simulink model "generic"  (R2022b)
settings: Solver=VariableStepAuto  StartTime=0.0  StopTime=inf  RelTol=1e-3
undefined symbols (not defined in the file or in its folder): left_first_line_point_x, right_first_line_point_x, route1_waypoint_raw
libraries: CarMaker4SL x69, slpidlib x3, simulink x1
(part 3 of 4)

== system generic/CarMaker/IPG Vehicle/CarAndTrailer/Forces/Vehicle Forces ==
  Sync_In : Inport
  Bus Creator1 : BusCreator  Inputs=12
  Bus Creator8 : BusCreator  Inputs=16
  BusCreator1 : BusCreator  Inputs=4
  BusCreator2 : BusCreator  Inputs=9
  Demux : Demux  Outputs=16
      settings: DisplayOption=none
  Demux1 : Demux  Outputs=12
      settings: DisplayOption=none
  Demux2 : Demux  Outputs=13
      settings: DisplayOption=none
  Forces : S-Function  FunctionName=CM_Sfun  Parameters='Forces'  SFunctionDeploymentMode=off  EnableBusSupport=off
  Terminator : Terminator
  Sync_Out : Outport  VectorParamsAs1DForOutWhenUnconnected=off
  Car.Virtual : Outport  Port=2  VectorParamsAs1DForOutWhenUnconnected=off
  Car.Aero : Outport  Port=3  VectorParamsAs1DForOutWhenUnconnected=off
  Car.Load : Outport  Port=4  VectorParamsAs1DForOutWhenUnconnected=off
  wires:
  BusCreator1/1 -> Terminator/1  "Aero IF (in)"
  Demux2/13 -> BusCreator2/9  "car Aero Trq_1 z"
  Demux2/12 -> BusCreator2/8  "car Aero Trq_1 y"
  Demux2/11 -> BusCreator2/7  "car Aero Trq_1 x"
  Demux2/10 -> BusCreator2/6  "car Aero Frc_1 z"
  Demux2/9 -> BusCreator2/5  "car Aero Frc_1 y"
  Demux2/8 -> BusCreator2/4  "car Aero Frc_1 x"
  Demux2/7 -> BusCreator2/3  "car Aero PoA_1 z"
  Demux2/6 -> BusCreator2/2  "car Aero PoA_1 y"
  Demux2/5 -> BusCreator2/1  "car Aero PoA_1 x"
  Demux2/4 -> BusCreator1/4  "car Aero tau_1"
  Demux2/3 -> BusCreator1/3  "car Aero ApproachVel_1 z"
  Demux2/2 -> BusCreator1/2  "car Aero ApproachVel_1 y"
  Demux2/1 -> BusCreator1/1  "car Aero ApproachVel_1 x"
  Demux/16 -> Bus Creator8/16  "Car Load_3 tz"
  Demux/15 -> Bus Creator8/15  "Car Load_3 ty"
  Demux/14 -> Bus Creator8/14  "Car Load_3 tx"
  Demux/13 -> Bus Creator8/13  "Car Load_3 mass"
  Demux1/12 -> Bus Creator1/12  "Car Virtual Trq_0 z"
  Demux1/11 -> Bus Creator1/11  "Car Virtual Trq_0 y"
  Demux1/10 -> Bus Creator1/10  "Car Virtual Trq_0 x"
  Demux1/9 -> Bus Creator1/9  "Car Virtual Trq_1 z"
  Demux1/8 -> Bus Creator1/8  "Car Virtual Trq_1 y"
  Demux1/7 -> Bus Creator1/7  "Car Virtual Trq_1 x"
  Demux1/6 -> Bus Creator1/6  "Car Virtual Frc_0 z"
  Demux1/5 -> Bus Creator1/5  "Car Virtual Frc_0 y"
  Demux1/4 -> Bus Creator1/4  "Car Virtual Frc_0 x"
  Sync_In/1 -> Forces/1
  Forces/1 -> Sync_Out/1
  BusCreator2/1 -> Car.Aero/1
  Demux1/1 -> Bus Creator1/1  "Car Virtual Frc_1 x"
  Demux1/2 -> Bus Creator1/2  "Car Virtual Frc_1 y"
  Demux1/3 -> Bus Creator1/3  "Car Virtual Frc_1 z"
  Forces/3 -> Demux2/1
  Forces/2 -> Demux1/1
  Bus Creator1/1 -> Car.Virtual/1
  Bus Creator8/1 -> Car.Load/1
  Demux/1 -> Bus Creator8/1  "Car Load_0 mass"
  Demux/2 -> Bus Creator8/2  "Car Load_0 tx"
  Demux/3 -> Bus Creator8/3  "Car Load_0 ty"
  Demux/4 -> Bus Creator8/4  "Car Load_0 tz"
  Demux/5 -> Bus Creator8/5  "Car Load_1 mass"
  Demux/6 -> Bus Creator8/6  "Car Load_1 tx"
  Demux/7 -> Bus Creator8/7  "Car Load_1 ty"
  Demux/8 -> Bus Creator8/8  "Car Load_1 tz"
  Demux/9 -> Bus Creator8/9  "Car Load_2 mass"
  Demux/10 -> Bus Creator8/10  "Car Load_2 tx"
  Demux/11 -> Bus Creator8/11  "Car Load_2 ty"
  Demux/12 -> Bus Creator8/12  "Car Load_2 tz"
  Forces/4 -> Demux/1

== system generic/CarMaker/IPG Vehicle/CarAndTrailer/Trailer/CreateBus Car.Hitch.FrcTrq ==
  In1 : Inport
  Bus Creator7 : BusCreator  Inputs=6
  Demux7 : Demux  Outputs=6
      settings: DisplayOption=none
  Out1 : Outport  VectorParamsAs1DForOutWhenUnconnected=off
  wires:
  In1/1 -> Demux7/1
  Bus Creator7/1 -> Out1/1
  Demux7/6 -> Bus Creator7/6  "Car Hitch Trq2Car z"
  Demux7/5 -> Bus Creator7/5  "Car Hitch Trq2Car y"
  Demux7/4 -> Bus Creator7/4  "Car Hitch Trq2Car x"
  Demux7/3 -> Bus Creator7/3  "Car Hitch Frc2Car z"
  Demux7/2 -> Bus Creator7/2  "Car Hitch Frc2Car y"
  Demux7/1 -> Bus Creator7/1  "Car Hitch Frc2Car x"

== system generic/CarMaker/IPG Vehicle/CarAndTrailer/Trailer/CreateBus Vhcl.Motion ==
  In1 : Inport
  BusCreator : BusCreator  Inputs=15
  Demux : Demux  Outputs=15
      settings: DisplayOption=none
  Out1 : Outport  VectorParamsAs1DForOutWhenUnconnected=off
  wires:
  Demux/15 -> BusCreator/15  "Vhcl YawAcc"
  Demux/14 -> BusCreator/14  "Vhcl YawVel"
  Demux/13 -> BusCreator/13  "Vhcl Yaw"
  Demux/12 -> BusCreator/12  "Vhcl PitchAcc"
  Demux/11 -> BusCreator/11  "Vhcl PitchVel"
  Demux/10 -> BusCreator/10  "Vhcl Pitch"
  Demux/9 -> BusCreator/9  "Vhcl RollAcc"
  Demux/8 -> BusCreator/8  "Vhcl RollVel"
  Demux/7 -> BusCreator/7  "Vhcl Roll"
  Demux/6 -> BusCreator/6  "Vhcl Hitch_Pos z"
  Demux/5 -> BusCreator/5  "Vhcl Hitch_Pos y"
  Demux/4 -> BusCreator/4  "Vhcl Hitch_Pos x"
  Demux/3 -> BusCreator/3  "Vhcl sRoad"
  Demux/2 -> BusCreator/2  "Vhcl Distance"
  Demux/1 -> BusCreator/1  "Vhcl v"
  In1/1 -> Demux/1
  BusCreator/1 -> Out1/1

== system generic/CarMaker/IPG Vehicle/CarAndTrailer/Trailer/CreateBus Vhcl.PoI ==
  In1 : Inport
  Bus Creator3 : BusCreator  Inputs=18
  Demux3 : Demux  Outputs=18
      settings: DisplayOption=none
  Out1 : Outport  VectorParamsAs1DForOutWhenUnconnected=off
  wires:
  Demux3/18 -> Bus Creator3/18  "Vhcl PoI_GCS Elev"
  Demux3/17 -> Bus Creator3/17  "Vhcl PoI_GCS Lat"
  Demux3/16 -> Bus Creator3/16  "Vhcl PoI_GCS Long"
  Demux3/15 -> Bus Creator3/15  "Vhcl PoI_Acc_1 z"
  Demux3/14 -> Bus Creator3/14  "Vhcl PoI_Acc_1 y"
  Demux3/13 -> Bus Creator3/13  "Vhcl PoI_Acc_1 x"
  Demux3/12 -> Bus Creator3/12  "Vhcl PoI_Vel_1 z"
  Demux3/11 -> Bus Creator3/11  "Vhcl PoI_Vel_1 y"
  Demux3/10 -> Bus Creator3/10  "Vhcl PoI_Vel_1 x"
  Demux3/9 -> Bus Creator3/9  "Vhcl PoI_Acc z"
  Demux3/8 -> Bus Creator3/8  "Vhcl PoI_Acc y"
  Demux3/7 -> Bus Creator3/7  "Vhcl PoI_Acc x"
  Demux3/6 -> Bus Creator3/6  "Vhcl PoI_Vel z"
  Demux3/5 -> Bus Creator3/5  "Vhcl PoI_Vel y"
  Demux3/4 -> Bus Creator3/4  "Vhcl PoI_Vel x"
  Demux3/3 -> Bus Creator3/3  "Vhcl PoI_Pos z"
  Demux3/2 -> Bus Creator3/2  "Vhcl PoI_Pos y"
  In1/1 -> Demux3/1
  Bus Creator3/1 -> Out1/1
  Demux3/1 -> Bus Creator3/1  "Vhcl PoI_Pos x"

== system generic/CarMaker/IPG Vehicle/CarAndTrailer/Trailer/CreateBus Vhcl.Steering ==
  In1 : Inport
  Bus Creator3 : BusCreator  Inputs=4
  Demux : Demux
      settings: DisplayOption=none
  Out1 : Outport  VectorParamsAs1DForOutWhenUnconnected=off
  wires:
  Bus Creator3/1 -> Out1/1
  Demux/1 -> Bus Creator3/1  "Vhcl Steering Ang"
  Demux/3 -> Bus Creator3/3  "Vhcl Steering AngAcc"
  Demux/2 -> Bus Creator3/2  "Vhcl Steering AngVel"
  Demux/4 -> Bus Creator3/4  "Vhcl Steering Trq"
  In1/1 -> Demux/1

== system generic/CarMaker/IPG Vehicle/CarAndTrailer/Trailer/CreateBus Vhcl.Wheel.FL ==
  In1 : Inport
  Bus Creator3 : BusCreator  Inputs=14
  Demux3 : Demux  Outputs=14
      settings: DisplayOption=none
  Out1 : Outport  VectorParamsAs1DForOutWhenUnconnected=off
  wires:
  Demux3/14 -> Bus Creator3/14  "Vhcl Wheel FL Trq_WhlBearing"
  Demux3/13 -> Bus Creator3/13  "Vhcl Wheel FL Trq_T2W"
  Demux3/12 -> Bus Creator3/12  "Vhcl Wheel FL SideSlip"
  Demux3/11 -> Bus Creator3/11  "Vhcl Wheel FL LongSlip"
  Demux3/10 -> Bus Creator3/10  "Vhcl Wheel FL vBelt"
  Demux3/9 -> Bus Creator3/9  "Vhcl Wheel FL Fz"
  Demux3/8 -> Bus Creator3/8  "Vhcl Wheel FL Fy"
  Demux3/7 -> Bus Creator3/7  "Vhcl Wheel FL Fx"
  Demux3/6 -> Bus Creator3/6  "Vhcl Wheel FL r_zxy z"
  Demux3/5 -> Bus Creator3/5  "Vhcl Wheel FL r_zxy y"
  Demux3/4 -> Bus Creator3/4  "Vhcl Wheel FL r_zxy x"
  Demux3/3 -> Bus Creator3/3  "Vhcl Wheel FL t z"
  Demux3/2 -> Bus Creator3/2  "Vhcl Wheel FL t y"
  In1/1 -> Demux3/1
  Bus Creator3/1 -> Out1/1
  Demux3/1 -> Bus Creator3/1  "Vhcl Wheel FL t x"

== system generic/CarMaker/IPG Vehicle/CarAndTrailer/Trailer/CreateBus Vhcl.Wheel.FR ==
  In1 : Inport
  Bus Creator3 : BusCreator  Inputs=14
  Demux3 : Demux  Outputs=14
      settings: DisplayOption=none
  Out1 : Outport  VectorParamsAs1DForOutWhenUnconnected=off
  wires:
  Demux3/14 -> Bus Creator3/14  "Vhcl Wheel FR Trq_WhlBearing"
  Demux3/13 -> Bus Creator3/13  "Vhcl Wheel FR Trq_T2W"
  Demux3/12 -> Bus Creator3/12  "Vhcl Wheel FR SideSlip"
  Demux3/11 -> Bus Creator3/11  "Vhcl Wheel FR LongSlip"
  Demux3/10 -> Bus Creator3/10  "Vhcl Wheel FR vBelt"
  Demux3/9 -> Bus Creator3/9  "Vhcl Wheel FR Fz"
  Demux3/8 -> Bus Creator3/8  "Vhcl Wheel FR Fy"
  Demux3/7 -> Bus Creator3/7  "Vhcl Wheel FR Fx"
  Demux3/6 -> Bus Creator3/6  "Vhcl Wheel FR r_zxy z"
  Demux3/5 -> Bus Creator3/5  "Vhcl Wheel FR r_zxy y"
  Demux3/4 -> Bus Creator3/4  "Vhcl Wheel FR r_zxy x"
  Demux3/3 -> Bus Creator3/3  "Vhcl Wheel FR t z"
  Demux3/2 -> Bus Creator3/2  "Vhcl Wheel FR t y"
  In1/1 -> Demux3/1
  Bus Creator3/1 -> Out1/1
  Demux3/1 -> Bus Creator3/1  "Vhcl Wheel FR t x"

== system generic/CarMaker/IPG Vehicle/CarAndTrailer/Trailer/CreateBus Vhcl.Wheel.RL ==
  In1 : Inport
  Bus Creator3 : BusCreator  Inputs=14
  Demux3 : Demux  Outputs=14
      settings: DisplayOption=none
  Out1 : Outport  VectorParamsAs1DForOutWhenUnconnected=off
  wires:
  Demux3/14 -> Bus Creator3/14  "Vhcl Wheel RL Trq_WhlBearing"
  Demux3/13 -> Bus Creator3/13  "Vhcl Wheel RL Trq_T2W"
  Demux3/12 -> Bus Creator3/12  "Vhcl Wheel RL SideSlip"
  Demux3/11 -> Bus Creator3/11  "Vhcl Wheel RL LongSlip"
  Demux3/10 -> Bus Creator3/10  "Vhcl Wheel RL vBelt"
  Demux3/9 -> Bus Creator3/9  "Vhcl Wheel RL Fz"
  Demux3/8 -> Bus Creator3/8  "Vhcl Wheel RL Fy"
  Demux3/7 -> Bus Creator3/7  "Vhcl Wheel RL Fx"
  Demux3/6 -> Bus Creator3/6  "Vhcl Wheel RL r_zxy z"
  Demux3/5 -> Bus Creator3/5  "Vhcl Wheel RL r_zxy y"
  Demux3/4 -> Bus Creator3/4  "Vhcl Wheel RL r_zxy x"
  Demux3/3 -> Bus Creator3/3  "Vhcl Wheel RL t z"
  Demux3/2 -> Bus Creator3/2  "Vhcl Wheel RL t y"
  In1/1 -> Demux3/1
  Bus Creator3/1 -> Out1/1
  Demux3/1 -> Bus Creator3/1  "Vhcl Wheel RL t x"

== system generic/CarMaker/IPG Vehicle/CarAndTrailer/Trailer/CreateBus Vhcl.Wheel.RR ==
  In1 : Inport
  Bus Creator3 : BusCreator  Inputs=14
  Demux3 : Demux  Outputs=14
      settings: DisplayOption=none
  Out1 : Outport  VectorParamsAs1DForOutWhenUnconnected=off
  wires:
  Demux3/14 -> Bus Creator3/14  "Vhcl Wheel RR Trq_WhlBearing"
  Demux3/13 -> Bus Creator3/13  "Vhcl Wheel RR Trq_T2W"
  Demux3/12 -> Bus Creator3/12  "Vhcl Wheel RR SideSlip"
  Demux3/11 -> Bus Creator3/11  "Vhcl Wheel RR LongSlip"
  Demux3/10 -> Bus Creator3/10  "Vhcl Wheel RR vBelt"
  Demux3/9 -> Bus Creator3/9  "Vhcl Wheel RR Fz"
  Demux3/8 -> Bus Creator3/8  "Vhcl Wheel RR Fy"
  Demux3/7 -> Bus Creator3/7  "Vhcl Wheel RR Fx"
  Demux3/6 -> Bus Creator3/6  "Vhcl Wheel RR r_zxy z"
  Demux3/5 -> Bus Creator3/5  "Vhcl Wheel RR r_zxy y"
  Demux3/4 -> Bus Creator3/4  "Vhcl Wheel RR r_zxy x"
  Demux3/3 -> Bus Creator3/3  "Vhcl Wheel RR t z"
  Demux3/2 -> Bus Creator3/2  "Vhcl Wheel RR t y"
  In1/1 -> Demux3/1
  Bus Creator3/1 -> Out1/1
  Demux3/1 -> Bus Creator3/1  "Vhcl Wheel RR t x"

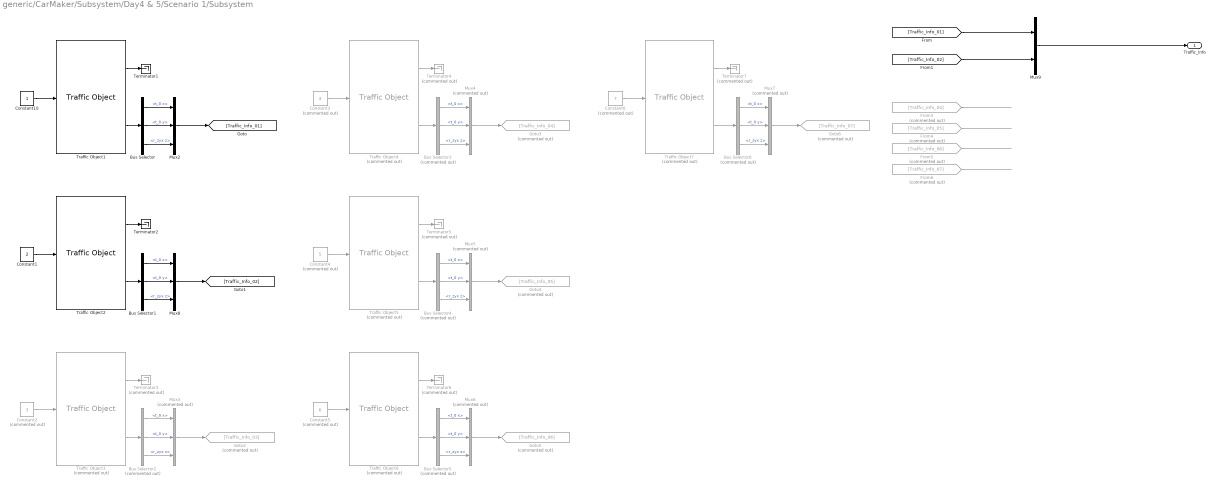
== system generic/CarMaker/Subsystem/Day4 & 5/Scenario 1/Subsystem ==
  Bus Selector : BusSelector  OutputSignals=t_0 x,t_0 y,r_zyx z
  Bus Selector1 : BusSelector  OutputSignals=t_0 x,t_0 y,r_zyx z
  Bus Selector{2..6} (5 alike) : BusSelector  Commented=on  OutputSignals=t_0 x,t_0 y,r_zyx z
  Constant1 : Constant  Value=2
  Constant10 : Constant
  Constant2 : Constant  Commented=on  Value=3
  Constant3 : Constant  Commented=on  Value=4
  Constant4 : Constant  Commented=on  Value=5
  Constant5 : Constant  Commented=on  Value=6
  Constant6 : Constant  Commented=on  Value=7
  From3 : From  Commented=on  GotoTag=Traffic_Info_04
  From4 : From  Commented=on  GotoTag=Traffic_Info_05
  From5 : From  Commented=on  GotoTag=Traffic_Info_06
  From6 : From  Commented=on  GotoTag=Traffic_Info_07
  Goto2 : Goto  Commented=on  GotoTag=Traffic_Info_03
  Goto3 : Goto  Commented=on  GotoTag=Traffic_Info_04
  Goto4 : Goto  Commented=on  GotoTag=Traffic_Info_05
  Goto5 : Goto  Commented=on  GotoTag=Traffic_Info_06
  Goto6 : Goto  Commented=on  GotoTag=Traffic_Info_07
  Mux2 : Mux  Inputs=3
  Mux{3..7} (5 alike) : Mux  Commented=on  Inputs=3
  Mux8 : Mux  Inputs=3
  Mux9 : Mux  Inputs=2
  Terminator1 : Terminator
  Terminator2 : Terminator
  Terminator{3..7} (5 alike) : Terminator  Commented=on
  Traffic Object1 : CarMaker4SL/Traffic Object  xname=T01  ximode=Traffic Id  xstime=Inherited
      settings: SourceProductName=CarMaker4SL
  Traffic Object2 : CarMaker4SL/Traffic Object  xname=T02  ximode=Traffic Id  xstime=Inherited
      settings: SourceProductName=CarMaker4SL
  Traffic Object3 : CarMaker4SL/Traffic Object  Commented=on  xname=T03  ximode=Traffic Id  xstime=Inherited
      settings: SourceProductName=CarMaker4SL
  Traffic Object4 : CarMaker4SL/Traffic Object  Commented=on  xname=T04  ximode=Traffic Id  xstime=Inherited
      settings: SourceProductName=CarMaker4SL
  Traffic Object5 : CarMaker4SL/Traffic Object  Commented=on  xname=T05  ximode=Traffic Id  xstime=Inherited
      settings: SourceProductName=CarMaker4SL
  Traffic Object6 : CarMaker4SL/Traffic Object  Commented=on  xname=T06  ximode=Traffic Id  xstime=Inherited
      settings: SourceProductName=CarMaker4SL
  Traffic Object7 : CarMaker4SL/Traffic Object  Commented=on  xname=T07  ximode=Traffic Id  xstime=Inherited
      settings: SourceProductName=CarMaker4SL
  Traffic_Info : Outport
  wires:
  Constant10/1 -> Traffic Object1/1
  Traffic Object1/1 -> Terminator1/1
  Traffic Object2/1 -> Terminator2/1
  Constant1/1 -> Traffic Object2/1
  Constant2/1 -> Traffic Object3/1
  Traffic Object3/1 -> Terminator3/1
  Traffic Object4/1 -> Terminator4/1
  Constant3/1 -> Traffic Object4/1
  Constant4/1 -> Traffic Object5/1
  Traffic Object5/1 -> Terminator5/1
  Traffic Object6/1 -> Terminator6/1
  Constant5/1 -> Traffic Object6/1
  Constant6/1 -> Traffic Object7/1
  Traffic Object7/1 -> Terminator7/1
  From3/1 -> ?
  From4/1 -> ?
  From5/1 -> ?
  From6/1 -> ?
  Traffic Object1/2 -> Bus Selector/1
  Bus Selector/1 -> Mux2/1  "<t_0 x>"
  Bus Selector/2 -> Mux2/2  "<t_0 y>"
  Bus Selector/3 -> Mux2/3  "<r_zyx z>"
  Bus Selector1/2 -> Mux8/2  "<t_0 y>"
  Mux8/1 -> [Traffic_Info_02]
  Bus Selector1/1 -> Mux8/1  "<t_0 x>"
  Bus Selector1/3 -> Mux8/3  "<r_zyx z>"
  Traffic Object2/2 -> Bus Selector1/1
  Bus Selector2/2 -> Mux3/2  "<t_0 y>"
  Mux3/1 -> Goto2/1
  Bus Selector2/1 -> Mux3/1  "<t_0 x>"
  Bus Selector2/3 -> Mux3/3  "<r_zyx z>"
  Traffic Object3/2 -> Bus Selector2/1
  Bus Selector3/2 -> Mux4/2  "<t_0 y>"
  Mux4/1 -> Goto3/1
  Bus Selector3/1 -> Mux4/1  "<t_0 x>"
  Bus Selector3/3 -> Mux4/3  "<r_zyx z>"
  Traffic Object4/2 -> Bus Selector3/1
  Bus Selector4/2 -> Mux5/2  "<t_0 y>"
  Mux5/1 -> Goto4/1
  Bus Selector4/1 -> Mux5/1  "<t_0 x>"
  Bus Selector4/3 -> Mux5/3  "<r_zyx z>"
  Traffic Object5/2 -> Bus Selector4/1
  Bus Selector5/2 -> Mux6/2  "<t_0 y>"
  Mux6/1 -> Goto5/1
  Bus Selector5/1 -> Mux6/1  "<t_0 x>"
  Bus Selector5/3 -> Mux6/3  "<r_zyx z>"
  Traffic Object6/2 -> Bus Selector5/1
  Bus Selector6/2 -> Mux7/2  "<t_0 y>"
  Mux7/1 -> Goto6/1
  Bus Selector6/1 -> Mux7/1  "<t_0 x>"
  Bus Selector6/3 -> Mux7/3  "<r_zyx z>"
  Traffic Object7/2 -> Bus Selector6/1
  Mux2/1 -> [Traffic_Info_01]
  [Traffic_Info_01] -> Mux9/1
  [Traffic_Info_02] -> Mux9/2
  Mux9/1 -> Traffic_Info/1

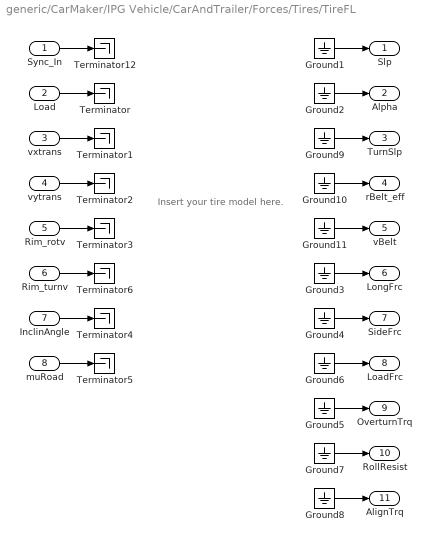
== system generic/CarMaker/IPG Vehicle/CarAndTrailer/Forces/Tires/TireFL ==
  note: Insert your tire model here.
  Sync_In : Inport
  Load : Inport  Port=2
  vxtrans : Inport  Port=3
  vytrans : Inport  Port=4
  Rim_rotv : Inport  Port=5
  Rim_turnv : Inport  Port=6
  InclinAngle : Inport  Port=7
  muRoad : Inport  Port=8
  Ground{1..11} (11 alike) : Ground
  Terminator{,1..6,12} (8 alike) : Terminator
  Slp : Outport  VectorParamsAs1DForOutWhenUnconnected=off
  Alpha : Outport  Port=2  VectorParamsAs1DForOutWhenUnconnected=off
  TurnSlp : Outport  Port=3  VectorParamsAs1DForOutWhenUnconnected=off
  rBelt_eff : Outport  Port=4  VectorParamsAs1DForOutWhenUnconnected=off
  vBelt : Outport  Port=5  VectorParamsAs1DForOutWhenUnconnected=off
  LongFrc : Outport  Port=6  VectorParamsAs1DForOutWhenUnconnected=off
  SideFrc : Outport  Port=7  VectorParamsAs1DForOutWhenUnconnected=off
  LoadFrc : Outport  Port=8  VectorParamsAs1DForOutWhenUnconnected=off
  OverturnTrq : Outport  Port=9  VectorParamsAs1DForOutWhenUnconnected=off
  RollResist : Outport  Port=10  VectorParamsAs1DForOutWhenUnconnected=off
  AlignTrq : Outport  Port=11  VectorParamsAs1DForOutWhenUnconnected=off
  wires:
  Ground11/1 -> vBelt/1
  Ground10/1 -> rBelt_eff/1
  Ground9/1 -> TurnSlp/1
  Rim_turnv/1 -> Terminator6/1
  Sync_In/1 -> Terminator12/1
  Ground2/1 -> Alpha/1
  Ground3/1 -> LongFrc/1
  Ground4/1 -> SideFrc/1
  Ground5/1 -> OverturnTrq/1
  vxtrans/1 -> Terminator1/1
  vytrans/1 -> Terminator2/1
  Rim_rotv/1 -> Terminator3/1
  InclinAngle/1 -> Terminator4/1
  muRoad/1 -> Terminator5/1
  Load/1 -> Terminator/1
  Ground1/1 -> Slp/1
  Ground6/1 -> LoadFrc/1
  Ground7/1 -> RollResist/1
  Ground8/1 -> AlignTrq/1

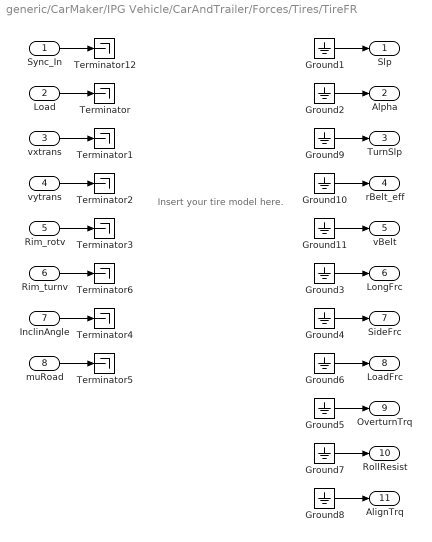
== system generic/CarMaker/IPG Vehicle/CarAndTrailer/Forces/Tires/TireFR ==
  note: Insert your tire model here.
  Sync_In : Inport
  Load : Inport  Port=2
  vxtrans : Inport  Port=3
  vytrans : Inport  Port=4
  Rim_rotv : Inport  Port=5
  Rim_turnv : Inport  Port=6
  InclinAngle : Inport  Port=7
  muRoad : Inport  Port=8
  Ground{1..11} (11 alike) : Ground
  Terminator{,1..6,12} (8 alike) : Terminator
  Slp : Outport  VectorParamsAs1DForOutWhenUnconnected=off
  Alpha : Outport  Port=2  VectorParamsAs1DForOutWhenUnconnected=off
  TurnSlp : Outport  Port=3  VectorParamsAs1DForOutWhenUnconnected=off
  rBelt_eff : Outport  Port=4  VectorParamsAs1DForOutWhenUnconnected=off
  vBelt : Outport  Port=5  VectorParamsAs1DForOutWhenUnconnected=off
  LongFrc : Outport  Port=6  VectorParamsAs1DForOutWhenUnconnected=off
  SideFrc : Outport  Port=7  VectorParamsAs1DForOutWhenUnconnected=off
  LoadFrc : Outport  Port=8  VectorParamsAs1DForOutWhenUnconnected=off
  OverturnTrq : Outport  Port=9  VectorParamsAs1DForOutWhenUnconnected=off
  RollResist : Outport  Port=10  VectorParamsAs1DForOutWhenUnconnected=off
  AlignTrq : Outport  Port=11  VectorParamsAs1DForOutWhenUnconnected=off
  wires:
  Ground11/1 -> vBelt/1
  Ground10/1 -> rBelt_eff/1
  Ground9/1 -> TurnSlp/1
  Rim_turnv/1 -> Terminator6/1
  Sync_In/1 -> Terminator12/1
  Ground2/1 -> Alpha/1
  Ground3/1 -> LongFrc/1
  Ground4/1 -> SideFrc/1
  Ground5/1 -> OverturnTrq/1
  vxtrans/1 -> Terminator1/1
  vytrans/1 -> Terminator2/1
  Rim_rotv/1 -> Terminator3/1
  InclinAngle/1 -> Terminator4/1
  muRoad/1 -> Terminator5/1
  Load/1 -> Terminator/1
  Ground1/1 -> Slp/1
  Ground6/1 -> LoadFrc/1
  Ground7/1 -> RollResist/1
  Ground8/1 -> AlignTrq/1

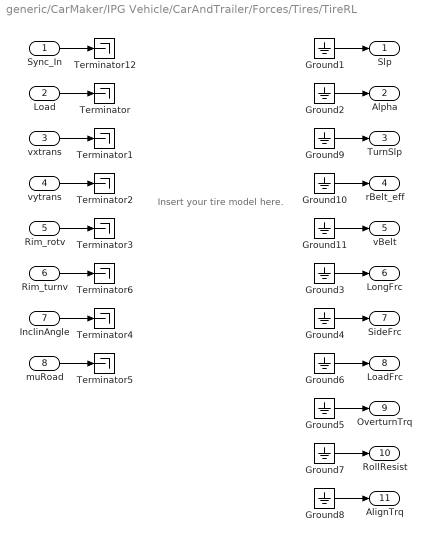
== system generic/CarMaker/IPG Vehicle/CarAndTrailer/Forces/Tires/TireRL ==
  note: Insert your tire model here.
  Sync_In : Inport
  Load : Inport  Port=2
  vxtrans : Inport  Port=3
  vytrans : Inport  Port=4
  Rim_rotv : Inport  Port=5
  Rim_turnv : Inport  Port=6
  InclinAngle : Inport  Port=7
  muRoad : Inport  Port=8
  Ground{1..11} (11 alike) : Ground
  Terminator{,1..6,12} (8 alike) : Terminator
  Slp : Outport  VectorParamsAs1DForOutWhenUnconnected=off
  Alpha : Outport  Port=2  VectorParamsAs1DForOutWhenUnconnected=off
  TurnSlp : Outport  Port=3  VectorParamsAs1DForOutWhenUnconnected=off
  rBelt_eff : Outport  Port=4  VectorParamsAs1DForOutWhenUnconnected=off
  vBelt : Outport  Port=5  VectorParamsAs1DForOutWhenUnconnected=off
  LongFrc : Outport  Port=6  VectorParamsAs1DForOutWhenUnconnected=off
  SideFrc : Outport  Port=7  VectorParamsAs1DForOutWhenUnconnected=off
  LoadFrc : Outport  Port=8  VectorParamsAs1DForOutWhenUnconnected=off
  OverturnTrq : Outport  Port=9  VectorParamsAs1DForOutWhenUnconnected=off
  RollResist : Outport  Port=10  VectorParamsAs1DForOutWhenUnconnected=off
  AlignTrq : Outport  Port=11  VectorParamsAs1DForOutWhenUnconnected=off
  wires:
  Ground11/1 -> vBelt/1
  Ground10/1 -> rBelt_eff/1
  Ground9/1 -> TurnSlp/1
  Rim_turnv/1 -> Terminator6/1
  Sync_In/1 -> Terminator12/1
  Ground2/1 -> Alpha/1
  Ground3/1 -> LongFrc/1
  Ground4/1 -> SideFrc/1
  Ground5/1 -> OverturnTrq/1
  vxtrans/1 -> Terminator1/1
  vytrans/1 -> Terminator2/1
  Rim_rotv/1 -> Terminator3/1
  InclinAngle/1 -> Terminator4/1
  muRoad/1 -> Terminator5/1
  Load/1 -> Terminator/1
  Ground1/1 -> Slp/1
  Ground6/1 -> LoadFrc/1
  Ground7/1 -> RollResist/1
  Ground8/1 -> AlignTrq/1

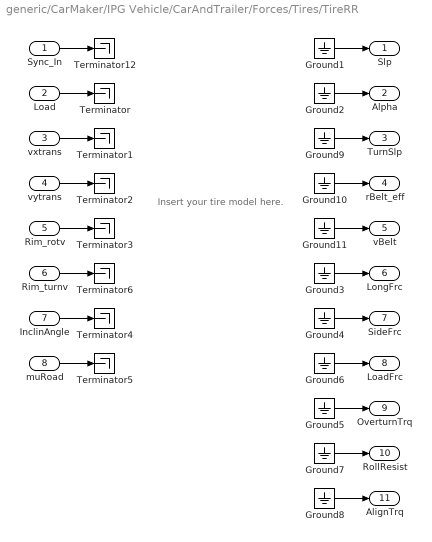
== system generic/CarMaker/IPG Vehicle/CarAndTrailer/Forces/Tires/TireRR ==
  note: Insert your tire model here.
  Sync_In : Inport
  Load : Inport  Port=2
  vxtrans : Inport  Port=3
  vytrans : Inport  Port=4
  Rim_rotv : Inport  Port=5
  Rim_turnv : Inport  Port=6
  InclinAngle : Inport  Port=7
  muRoad : Inport  Port=8
  Ground{1..11} (11 alike) : Ground
  Terminator{,1..6,12} (8 alike) : Terminator
  Slp : Outport  VectorParamsAs1DForOutWhenUnconnected=off
  Alpha : Outport  Port=2  VectorParamsAs1DForOutWhenUnconnected=off
  TurnSlp : Outport  Port=3  VectorParamsAs1DForOutWhenUnconnected=off
  rBelt_eff : Outport  Port=4  VectorParamsAs1DForOutWhenUnconnected=off
  vBelt : Outport  Port=5  VectorParamsAs1DForOutWhenUnconnected=off
  LongFrc : Outport  Port=6  VectorParamsAs1DForOutWhenUnconnected=off
  SideFrc : Outport  Port=7  VectorParamsAs1DForOutWhenUnconnected=off
  LoadFrc : Outport  Port=8  VectorParamsAs1DForOutWhenUnconnected=off
  OverturnTrq : Outport  Port=9  VectorParamsAs1DForOutWhenUnconnected=off
  RollResist : Outport  Port=10  VectorParamsAs1DForOutWhenUnconnected=off
  AlignTrq : Outport  Port=11  VectorParamsAs1DForOutWhenUnconnected=off
  wires:
  Ground11/1 -> vBelt/1
  Ground10/1 -> rBelt_eff/1
  Ground9/1 -> TurnSlp/1
  Rim_turnv/1 -> Terminator6/1
  Sync_In/1 -> Terminator12/1
  Ground2/1 -> Alpha/1
  Ground3/1 -> LongFrc/1
  Ground4/1 -> SideFrc/1
  Ground5/1 -> OverturnTrq/1
  vxtrans/1 -> Terminator1/1
  vytrans/1 -> Terminator2/1
  Rim_rotv/1 -> Terminator3/1
  InclinAngle/1 -> Terminator4/1
  muRoad/1 -> Terminator5/1
  Load/1 -> Terminator/1
  Ground1/1 -> Slp/1
  Ground6/1 -> LoadFrc/1
  Ground7/1 -> RollResist/1
  Ground8/1 -> AlignTrq/1

== matlab function generic/CarMaker/Subsystem/Day1/Scenario 1/MATLAB Function1 ==
  settings: updateMethod=DISCRETE  sampleTime=0.05
  data: u input; y output
function y = kalman_filter_(u)
    ;
end

== matlab function generic/CarMaker/Subsystem/Day1/Scenario 1/MATLAB Function2 ==
  settings: updateMethod=DISCRETE  sampleTime=0.05
  data: u input; y output
function y = average_filter_(u)
    ;
end

== matlab function generic/CarMaker/Subsystem/Day2/Scenario 4 & 5/MATLAB Function1 ==
  settings: updateMethod=DISCRETE  sampleTime=0.05
  data: poly_coeff input; lateral_error output; velocity input; lookahead_time input; x_lookahead output
function [lateral_error,x_lookahead] = compute_lateral_error(poly_coeff, velocity, lookahead_time)
    ;
end

== matlab function generic/CarMaker/Subsystem/Day1/Scenario 1/MATLAB Function3 ==
  settings: updateMethod=DISCRETE  sampleTime=0.05
  data: u input; y output
function y = lowpass_filter_(u)
    ;
end

== matlab function generic/CarMaker/Subsystem/Day2/Scenario 4 & 5/MATLAB Function3 ==
  settings: updateMethod=DISCRETE  sampleTime=0.05
  data: local_waypoints input; poly_coeff output
function poly_coeff = fit_polynomial_to_waypoints(local_waypoints)
    ;
end

== matlab function generic/CarMaker/Subsystem/Day2/Scenario 4 & 5/MATLAB Function4  ==
  settings: updateMethod=DISCRETE  sampleTime=0.05
  data: waypoints input; local_waypoints_ output; vehicle_position input; head input
function local_waypoints_ = global_to_local_waypoints(waypoints, vehicle_position, head)
    ;
end

== matlab function generic/CarMaker/Subsystem/Day1/Scenario 3 & 4/MATLAB Function2 ==
  settings: updateMethod=DISCRETE  sampleTime=0.05
  data: cross_track_error input; tire_angle output
function tire_angle = lateral_pd_controller_(cross_track_error)
    ;
end

== matlab function generic/CarMaker/Subsystem/Day2/Scenario 1/MATLAB Function2 ==
  settings: updateMethod=DISCRETE  sampleTime=0.05
  data: target_velocity input; desired_ax output; ego_velocity input
function desired_ax = longitudinal_speed_pd_controller_(target_velocity, ego_velocity)
    ;
end

== matlab function generic/CarMaker/Subsystem/Day2/Scenario 2 & 3/MATLAB Function2 ==
  settings: updateMethod=DISCRETE  sampleTime=0.05
  data: target_distance input; desired_ax output; clearance input
function desired_ax = longitudinal_space_pid_controller_(target_distance, clearance)
    ;
end

== stateflow chart generic/CarMaker/Subsystem/Day3/Chart ==
  (default) -> (junction 1)
  (junction 1) -> (junction 3) [order 1] : [i<99]
      | {i = i + 1;}
  (junction 1) -> (junction 7) [order 2] : {i=0;}
  (junction 3) -> (junction 5)
  (junction 5) -> (junction 7)
  (junction 7) -> (junction 10)
  (junction 10) -> (junction 12) [order 1] : [i > 50]
      | {do_Logic;}
  (junction 10) -> (junction 18) [order 2]
  (junction 12) -> (junction 16)
  (junction 16) -> (junction 18)
  (junction 18) -> (junction 21)
  data: i local =0
  events: do_Logic output FUNCTION_CALL_EVENT

== matlab function generic/CarMaker/Subsystem/Final Project/Scenario 1/MATLAB Function1 ==
  settings: updateMethod=DISCRETE  sampleTime=0.1
  data: u1 input; y output; u2 input
function y = longitudinal_speed_pd_controller_(u1, u2)
    ;
end

== matlab function generic/CarMaker/Subsystem/Day3/Triggered Subsystem/MATLAB Function4  ==
  settings: sampleTime=0.1
  data: waypoints_x input; waypoints_y input; local_waypoints_ output; vehicle_position input; head input; qual input; ego_idx_out output; ego_valid output
function [local_waypoints_,ego_idx_out,ego_valid]  = global_to_local_waypoints(waypoints_x,waypoints_y, vehicle_position, head, qual)
    ;
end

== matlab function generic/CarMaker/Subsystem/Day3/Triggered Subsystem/MATLAB Function4 1 ==
  settings: sampleTime=0.1
  data: waypoints_x input; waypoints_y input; local_waypoints_ output; vehicle_position input; head input; qual input; ego_idx_out output; ego_valid output
function [local_waypoints_,ego_idx_out,ego_valid]  = global_to_local_waypoints(waypoints_x,waypoints_y, vehicle_position, head, qual)
    ;
end

== matlab function generic/CarMaker/Subsystem/Day2/Scenario 2 & 3/MATLAB Function1 ==
  settings: updateMethod=DISCRETE  sampleTime=0.05
  data: ego_velocity input; desired_ax output; clearance input
function desired_ax = longitudinal_variant_space_pd_controller_(ego_velocity, clearance)
    ;
end

== matlab function generic/CarMaker/Subsystem/Final Project/Scenario 1/MATLAB Function2 ==
  settings: updateMethod=DISCRETE  sampleTime=0.1
  data: u input; y output
function y = lateral_pid_controller_(u)
    ;
end

== matlab function generic/CarMaker/Subsystem/Day4 & 5/Scenario 1/MATLAB Function1 ==
  settings: updateMethod=DISCRETE  sampleTime=0.05
  data: map_boundary input; mapMatrix output size=[1000, 1000]; traffic_info input; traffic_size input
function mapMatrix = generate_map_(map_boundary, traffic_info, traffic_size)
    ;
end

== matlab function generic/CarMaker/Subsystem/Day4 & 5/Scenario 1/MATLAB Function2 ==
  settings: updateMethod=DISCRETE  sampleTime=0.1
  data: map input; y output; traffic_info input; traffic_size input
function y = add_obstacle_(map, traffic_info, traffic_size)
    ;
end

== matlab function generic/CarMaker/Subsystem/Day6/Scenario 1/MATLAB Function1 ==
  settings: updateMethod=DISCRETE  sampleTime=0.1
  data: u1 input; y output; u2 input
function y = longitudinal_speed_pd_controller_(u1, u2)
    ;
end

== matlab function generic/CarMaker/Subsystem/Day6/Scenario 1/MATLAB Function2 ==
  settings: updateMethod=DISCRETE  sampleTime=0.1
  data: u input; y output
function y = lateral_pid_controller_(u)
    ;
end

== matlab function generic/CarMaker/Subsystem/Day3/Triggered Subsystem/MATLAB Function4 6 ==
  settings: sampleTime=0.1
  data: si input; si_d input; si_dd input; sf_d input; sf_dd input; di input; di_d input; di_dd input; df_d input; df_dd input; opt_d input; mapx input; mapy input; maps input; yaw_value output double size=[3,30]; s_d_value output double size=[3,30]
function [ yaw_value, s_d_value] = calc_frenet_and_global_paths(si, si_d, si_dd, sf_d, sf_dd, di, di_d, di_dd, df_d, df_dd, opt_d, mapx, mapy, maps)

    % Define constants
    TARGET_SPEED = 1;
    LANE_WIDTH = 0.39;
    DF_SET = [LANE_WIDTH/2, -LANE_WIDTH/2];
    MIN_T = 1; 
    MAX_T = 2; 
    DT_T = 1; 
    DT = 0.1; 
    MAX_POINTS = (MAX_T / DT) + 1;  % 사전 계산된 최대 포인트 수
    max_paths = length(DF_SET) * ((MAX_T - MIN_T) / DT_T + 1);

    % Cost weights
    K_J = 0.1; 
    K_T = 0.1; 
    K_D = 1.0; 
    K_V = 1.0; 
    K_LAT = 1.0; 
    K_LON = 1.0; 
    V_MAX = 2;        % Maximum velocity (example)
    ACC_MAX = 2;       % Maximum acceleration (example)
    K_MAX = 4;       % Maximum curvature (example)

    % Pre-allocate fixed-size struct array
    frenet_paths = repmat(initialize_frenet_path(MAX_POINTS), 1, max_paths);  % 고정 크기의 구조체 배열
    valid_paths = repmat(initialize_frenet_path(MAX_POINTS), 1, max_paths);  % 고정 크기 배열로 지정
    
    path_count = 1;  % Path index tracker
    valid_count = 1;  % Valid path index tracker

    % 각 lateral 목표로 경로 생성
    for df = DF_SET
        for T = MIN_T:DT_T:MAX_T
            if path_count > max_paths
                break;  % 최대 경로 수 초과 시 종료
            end
            
            % Initialize Frenet path struct
            fp = initialize_frenet_path(MAX_POINTS);

            % Quintic polynomial for lateral trajectory
            lat_traj = QuinticPolynomial(di, di_d, di_dd, df, df_d, df_dd, T);

            % Calculate lateral trajectory
            for i = 1:MAX_POINTS
                t = (i-1) * DT;
                if t > T
                    break;
                end
                fp.t(i) = t;
                fp.d(i) = lat_traj.calc_pos(t);
                fp.d_d(i) = lat_traj.calc_vel(t);
                fp.d_dd(i) = lat_traj.calc_acc(t);
                fp.d_ddd(i) = lat_traj.calc_jerk(t);
            end

            % Longitudinal motion planning
            lon_traj = QuarticPolynomial(si, si_d, si_dd, sf_d, sf_dd, T);

            % Calculate longitudinal trajectory
            for i = 1:MAX_POINTS
                t = fp.t(i);
                if t > T
                    break;
                end
                fp.s(i) = lon_traj.calc_pos(t);
                fp.s_d(i) = lon_traj.calc_vel(t);
                fp.s_dd(i) = lon_traj.calc_acc(t);
                fp.s_ddd(i) = lon_traj.calc_jerk(t);
            end

            % Calculate costs
            J_lat = sum(fp.d_ddd .^ 2);  % Lateral jerk
            J_lon = sum(fp.s_ddd .^ 2);  % Longitudinal jerk

            % Consistency cost
            d_diff = (fp.d(end) - opt_d) ^ 2;
            v_diff = (TARGET_SPEED - fp.s_d(end)) ^ 2;

            % Update costs
            fp.c_lat = K_J * J_lat + K_T * T + K_D * d_diff;
            fp.c_lon = K_J * J_lon + K_T * T + K_V * v_diff;
            fp.c_tot = K_LAT * fp.c_lat + K_LON * fp.c_lon;

            % ---- Global Path Conversion ----
            % Frenet 좌표에서 Global 좌표로 변환
            for i = 1:length(fp.s)
                s_s = fp.s(i);
                d_d = fp.d(i);
                [fp.x(i), fp.y(i),~] = get_cartesian(s_s, d_d, mapx, mapy, maps);
            end

            % Yaw와 ds(거리 차이) 계산
            for i = 1:length(fp.x) - 1
                dx = fp.x(i + 1) - fp.x(i);
                dy = fp.y(i + 1) - fp.y(i);
                fp.yaw(i) = atan2(dy, dx);    % 방향 각도 계산
                fp.ds(i) = hypot(dx, dy);     % 두 점 사이의 거리 계산
            end
            
            % Yaw와 ds의 마지막 값을 복사
            fp.yaw(MAX_POINTS) = fp.yaw(MAX_POINTS-1);   % 마지막 yaw 값 복사
            fp.ds(MAX_POINTS) = fp.ds(MAX_POINTS-1);     % 마지막 ds 값 복사

            % 곡률(kappa) 계산
            for i = 1:length(fp.yaw) - 1
                yaw_diff = fp.yaw(i + 1) - fp.yaw(i);
                yaw_diff = atan2(sin(yaw_diff), cos(yaw_diff));
                fp.kappa(i) = yaw_diff / fp.ds(i);    % 곡률 계산
            end

            % Store the Frenet path in the array
            frenet_paths(path_count) = fp;
            path_count = path_count + 1;
        end
    end
    
    % ---- Check Path Validity ----
    for i = 1:length(frenet_paths)
        fp = frenet_paths(i);
        acc_squared = abs(fp.s_dd .^ 2 + fp.d_dd .^ 2);
        
        if any(fp.s_d > V_MAX)  % Max speed check
            continue;
        elseif any(acc_squared > ACC_MAX ^ 2)  % Max acceleration check
            continue;
        elseif any(abs(fp.kappa) > K_MAX)  % Max curvature check
            continue;
        end
        
        % 유효한 경로를 valid_frenet_paths에 저장
        valid_paths(valid_count) = fp;
        valid_count = valid_count + 1;
    end
    
    % 유효한 경로까지만 반환
    valid_paths = valid_paths(1:valid_count - 1);

    % ---- Preallocation ----
    max_valid_paths = length(valid_paths);  % valid_paths의 최대 크기


    % 경로 수만큼 opt_traj를 사전 할당
    opt_traj = repmat(initialize_frenet_path(MAX_POINTS), 1, max_valid_paths);
    
    opt_count = 0;  % 최적 경로를 저장할 인덱스
    
    min_cost = inf;  % 최소 비용을 무한대로 초기화
    
    % 유효한 경로 중 최소 비용 경로 찾기
    for i = 1:max_valid_paths
        if valid_paths(i).c_tot < min_cost
            min_cost = valid_paths(i).c_tot;
            opt_count = opt_count + 1;  % 최적 경로 카운터 증가
            opt_traj(opt_count) = valid_paths(i);  % 최적 경로 저장
        end
    end
    
    % 실제로 채워진 opt_traj만 반환
    opt_traj = opt_traj(1:opt_count);  % 사용한 크기만큼 자르기

   
    % ---- Extract Global Coordinate Values ----
    if ~isempty(valid_paths)
        % ---- Extract Global Coordinate Values ----
        max_length = max(arrayfun(@(p) length(p.x), valid_paths));
    
        % 고정 크기의 NaN 배열 생성 (각 경로마다 max_length에 맞춘다)
        x_value = NaN(length(valid_paths), max_length);
        y_value = NaN(length(valid_paths), max_length);
        yaw_value = NaN(length(valid_paths), max_length);
        ds_value = NaN(length(valid_paths), max_length);
        kappa_value = NaN(length(valid_paths), max_length);
        s_d_value = NaN(length(valid_paths), max_length);  % s_d 값도 추가
    
        % 각 경로의 값을 고정 크기 배열에 채움
        for i = 1:length(valid_paths)
            path_len = length(valid_paths(i).x);
            
            % Global 좌표계 값들
            x_value(i, 1:path_len) = valid_paths(i).x;
            y_value(i, 1:path_len) = valid_paths(i).y;
            yaw_value(i, 1:path_len) = valid_paths(i).yaw;
            ds_value(i, 1:path_len) = valid_paths(i).ds;
            kappa_value(i, 1:path_len) = valid_paths(i).kappa;
            s_d_value(i, 1:path_len) = valid_paths(i).s_d;  % s_d 값 채우기
        end
    else
        % 유효한 경로가 없는 경우 빈 배열 반환
        x_value = [];
        y_value = [];
        yaw_value = [];
        ds_value = [];
        kappa_value = [];
        s_d_value = [];  % s_d 값 반환
    end
end





% Helper function to initialize FrenetPath with fixed-size arrays
function fp = initialize_frenet_path(max_points)
    % Pre-allocate fixed-size arrays for Frenet path
    fp.t = zeros(1, max_points);
    fp.d = zeros(1, max_points);
    fp.d_d = zeros(1, max_points);
    fp.d_dd = zeros(1, max_points);
    fp.d_ddd = zeros(1, max_points);
    fp.s = zeros(1, max_points);
    fp.s_d = zeros(1, max_points);
    fp.s_dd = zeros(1, max_points);
    fp.s_ddd = zeros(1, max_points);
    fp.c_lat = 0;
    fp.c_lon = 0;
    fp.c_tot = 0;
    fp.x = zeros(1, max_points);
    fp.y = zeros(1, max_points);
    fp.yaw = zeros(1, max_points);
    fp.ds = zeros(1, max_points);
    fp.kappa = zeros(1, max_points);
end


function quintic = QuinticPolynomial(xi, vi, ai, xf, vf, af, T)
    % Quintic Polynomial coefficients
    a0 = xi;
    a1 = vi;
    a2 = 0.5 * ai;

    A = [T^3, T^4, T^5;
         3*T^2, 4*T^3, 5*T^4;
         6*T, 12*T^2, 20*T^3];

    b = [xf - a0 - a1*T - a2*T^2;
         vf - a1 - 2*a2*T;
         af - 2*a2];

    x = A\b;  % Solve linear system

    a3 = x(1);
    a4 = x(2);
    a5 = x(3);

    % Return handles for functions
    quintic.calc_pos = @(t) (a0 + a1*t + a2*t^2 + a3*t^3 + a4*t^4 + a5*t^5);
    quintic.calc_vel = @(t) (a1 + 2*a2*t + 3*a3*t^2 + 4*a4*t^3 + 5*a5*t^4);
    quintic.calc_acc = @(t) (2*a2 + 6*a3*t + 12*a4*t^2 + 20*a5*t^3);
    quintic.calc_jerk = @(t) (6*a3 + 24*a4*t + 60*a5*t^2);
end

function quartic = QuarticPolynomial(xi, vi, ai, vf, af, T)
    % Quartic Polynomial coefficients
    a0 = xi;
    a1 = vi;
    a2 = 0.5 * ai;

    A = [3*T^2, 4*T^3;
         6*T, 12*T^2];

    b = [vf - a1 - 2*a2*T;
         af - 2*a2];

    x = A\b;  % Solve linear system

    a3 = x(1);
    a4 = x(2);

    % Return handles for functions
    quartic.calc_pos = @(t) (a0 + a1*t + a2*t^2 + a3*t^3 + a4*t^4);
    quartic.calc_vel = @(t) (a1 + 2*a2*t + 3*a3*t^2 + 4*a4*t^3);
    quartic.calc_acc = @(t) (2*a2 + 6*a3*t + 12*a4*t^2);
    quartic.calc_jerk = @(t) (6*a3 + 24*a4*t);
end

function [x,y,heading]  = get_cartesian(s, d, mapx, mapy, maps)
    prev_wp = 1;

    % s를 maps 길이 내에서 모듈로 연산
    s = mod(s, maps(end-1));

    % s보다 작은 prev_wp 찾기
    while (s > maps(prev_wp + 1)) && (prev_wp < length(maps) - 1)
        prev_wp = prev_wp + 1;
    end

    % 다음 waypoint 찾기
    next_wp = mod(prev_wp + 1, length(mapx));

    dx = mapx(next_wp) - mapx(prev_wp);
    dy = mapy(next_wp) - mapy(prev_wp);

    % 방향(heading) 계산 [rad]
    heading = atan2(dy, dx);

    % s를 따라 segment에서 x, y 좌표 계산
    seg_s = s - maps(prev_wp);

    seg_x = mapx(prev_wp) + seg_s * cos(heading);
    seg_y = mapy(prev_wp) + seg_s * sin(heading);

    % 수직 방향으로 변환 (90도)
    perp_heading = heading + pi / 2;
    x = seg_x + d * cos(perp_heading);
    y = seg_y + d * sin(perp_heading);
end

== matlab function generic/CarMaker/Subsystem/Day3/Triggered Subsystem/MATLAB Function4 7 ==
  settings: sampleTime=0.1
  data: x input; y input; mapx input; mapy input; frenet_s output double; frenet_d output double
function [frenet_s, frenet_d] = get_frenet(x, y, mapx, mapy)
    % 다음 경로점 계산
    next_wp = next_waypoint(x, y, mapx, mapy);
    
    prev_wp = max(next_wp - 1, 1);  % 경계 설정
    
    % 경로 벡터와 차량 위치 벡터 계산
    n_x = mapx(next_wp) - mapx(prev_wp);
    n_y = mapy(next_wp) - mapy(prev_wp);
    x_x = x - mapx(prev_wp);
    x_y = y - mapy(prev_wp);

    % 내적을 이용한 투영 벡터 계산
    denom = (n_x^2 + n_y^2);
    
    % 투영 계산 시 분모가 0이 되지 않도록 체크
    if denom == 0
        proj_norm = 0;
    else
        proj_norm = (x_x * n_x + x_y * n_y) / denom;
    end
    
    proj_x = mapx(prev_wp) + proj_norm * n_x;
    proj_y = mapy(prev_wp) + proj_norm * n_y;

    % Frenet d 값 계산
    frenet_d = get_dist(x, y, proj_x, proj_y);

    % 방향에 따른 부호 결정 (크로스 프로덕트)
    ego_vec = [x_x, x_y, 0];
    map_vec = [n_x, n_y, 0];
    d_cross = cross(ego_vec, map_vec);

    if d_cross(3) > 0
        frenet_d = -frenet_d;
    end

    % Frenet s 값 계산 (이전 웨이포인트까지의 거리 합산)
    frenet_s = 0;
    for i = 1:(prev_wp - 1)
        frenet_s = frenet_s + get_dist(mapx(i), mapy(i), mapx(i + 1), mapy(i + 1));
    end
    % 현재 웨이포인트에서 투영 좌표까지의 거리 추가
    frenet_s = frenet_s + get_dist(mapx(prev_wp), mapy(prev_wp), proj_x, proj_y);
    
end

function next_wp = next_waypoint(x, y, mapx, mapy)
    closest_wp = get_closest_waypoints(x, y, mapx, mapy);
    
    % 경계 처리: 마지막 웨이포인트에 도달하면 순환
    if closest_wp >= length(mapx)
        next_wp = 1;  % 경로가 순환하는 경우 첫 웨이포인트로 돌아가기
        return;
    end

    % 다음 웨이포인트 계산
    map_vec = [mapx(closest_wp + 1) - mapx(closest_wp), mapy(closest_wp + 1) - mapy(closest_wp)];
    ego_vec = [x - mapx(closest_wp), y - mapy(closest_wp)];

    direction = sign(dot(map_vec, ego_vec));

    if direction >= 0
        next_wp = closest_wp + 1;
    else
        next_wp = closest_wp;
    end
end

function closest_wp = get_closest_waypoints(x, y, mapx, mapy)
    min_len = Inf;
    closest_wp = 0;  % 웨이포인트는 1에서 시작

    for i = 1:length(mapx)
        dist = get_dist(x, y, mapx(i), mapy(i));
        if dist < min_len
            min_len = dist;
            closest_wp = i;
        end
    end
end

function dist = get_dist(x1, y1, x2, y2)
    % 두 좌표 간의 거리 계산
    dist = sqrt((x1 - x2)^2 + (y1 - y2)^2);
end

== matlab function generic/CarMaker/Subsystem/Day1/Scenario 2/MATLAB Function4 ==
  settings: updateMethod=DISCRETE  sampleTime=0.05
  data: u input; y output
function y = kalman_filter_(u)
    ;
end

== matlab function generic/CarMaker/Subsystem/Day1/Scenario 2/MATLAB Function5 ==
  settings: updateMethod=DISCRETE  sampleTime=0.05
  data: u input; y output
function y = average_filter_(u)
    ;
end

== matlab function generic/CarMaker/Subsystem/Day1/Scenario 2/MATLAB Function6 ==
  settings: updateMethod=DISCRETE  sampleTime=0.05
  data: u input; y output
function y = lowpass_filter_(u)
    ;
end

== matlab function generic/CarMaker/Subsystem/Day3/Triggered Subsystem/MATLAB Function4 8 ==
  settings: sampleTime=0.1
  data: waypoints_Left input; waypoints_Right input; mapx output; mapy output
function [mapx, mapy] = compute_center_path(waypoints_Left, waypoints_Right)
    % 중앙 경로 계산
    map_center = (waypoints_Left + waypoints_Right) / 2;
    
    % mapx, mapy 추출
    mapx = map_center(:, 1); % X 좌표
    mapy = map_center(:, 2); % Y 좌표
end

== matlab function generic/CarMaker/Subsystem/Day3/Triggered Subsystem/MATLAB Function4 2 ==
  settings: sampleTime=0.1
  data: local_waypoints input; poly_coeff output; x_local output; y_local output
function [poly_coeff,x_local,y_local] = fit_polynomial_to_waypoints(local_waypoints)
    ;
end

== matlab function generic/CarMaker/Subsystem/Day3/Triggered Subsystem/MATLAB Function4 3 ==
  settings: sampleTime=0.1
  data: local_waypoints input; poly_coeff output; x_local output; y_local output
function [poly_coeff,x_local,y_local] = fit_polynomial_to_waypoints(local_waypoints)
    ;
end

== matlab function generic/CarMaker/Subsystem/Day3/Triggered Subsystem/MATLAB Function4 4 ==
  settings: sampleTime=0.1
  data: coeff_L input; poly_coeff output; is_L output; is_R output; coeff_R input; qual_L input; qual_R input; ego_idx_L input; ego_idx_R input; ego_valid_L input; ego_valid_R input; state output; laneWidth output; coeff_L_out output; coeff_R_out output
function [poly_coeff,is_L,is_R,state,laneWidth,coeff_L_out,coeff_R_out] = make_line_to_path(coeff_L,coeff_R,qual_L,qual_R,ego_idx_L, ego_idx_R,ego_valid_L,ego_valid_R)
    ;
end

== matlab function generic/CarMaker/Subsystem/Day3/Triggered Subsystem/MATLAB Function4 5 ==
  settings: sampleTime=0.1
  data: poly_coeff input; lateral_error output; x_lookahead output; velocity input; lookahead_time input
function [lateral_error,x_lookahead] = compute_lateral_error(poly_coeff, velocity, lookahead_time)
    ;
end

== matlab function generic/CarMaker/Subsystem/Day3/Triggered Subsystem1/MATLAB Function4  ==
  settings: sampleTime=0.1
  data: waypoints_x input; waypoints_y input; local_point output; vehicle_position input; head input; dist output
function [local_point,dist]  = global_to_local_waypoints(waypoints_x,waypoints_y, vehicle_position, head)
    ;
end

== matlab function generic/CarMaker/Subsystem/Day3/Triggered Subsystem1/MATLAB Function4 1 ==
  settings: sampleTime=0.1
  data: ego_pos input; ego_heading input; ego_pos output; target_pos output; ego_heading output; steering_angle output
function [ego_pos, target_pos, ego_heading, steering_angle] = follow_target(ego_pos, ego_heading) ...
end
